simulink model "vip_ut"  (Simulink 8.1)
settings: Solver=FixedStepDiscrete  StartTime=0.0  StopTime=10.0  FixedStep=5E-3  RelTol=1e-3
libraries: siltestlib x17, idiada_lib x7, vip x1
settings Model: Creator=xsellart  LastModifiedBy=AT015555
settings DataIOCC: SignalLoggingSaveFormat=Dataset
settings OptimizationCC: ExpressionDepthLimit=128
settings DebuggingCC: FcnCallInpInsideContextMsg=EnableAllAsError
settings GRTTargetCC: CombineOutputUpdateFcns=on  GRTInterface=off

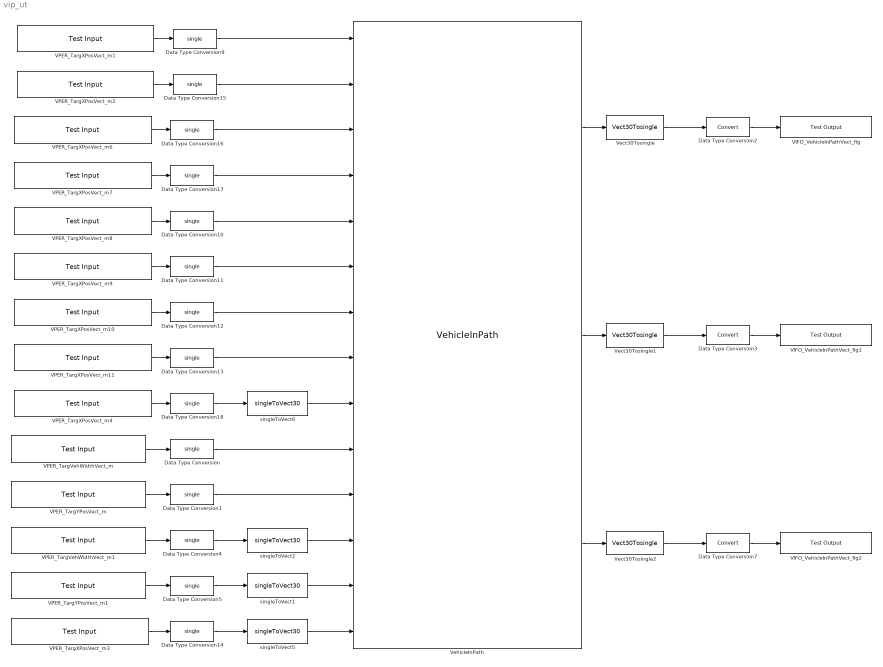
== system vip_ut ==
  Data Type Conversion{,1,4..5,9..18} (14 alike) : DataTypeConversion  OutDataTypeStr=single
  Data Type Conversion2 : DataTypeConversion
  Data Type Conversion3 : DataTypeConversion
  Data Type Conversion7 : DataTypeConversion
  VIFO_VehicleInPathVect_flg : siltestlib/Test Output  varname=VIFO_FCWVehInPathVect30_flg  sampletime=-1
  VIFO_VehicleInPathVect_flg1 : siltestlib/Test Output  varname=VIFO_AEBVehInPathVect30_flg  sampletime=-1
  VIFO_VehicleInPathVect_flg2 : siltestlib/Test Output  varname=VIFO_ACCVehInPathVect30_flg  sampletime=-1
  VPER_TargVehWidthVect_m : siltestlib/Test Input  varname=VDINR_YawRate_degps  sampletime=-1
  VPER_TargVehWidthVect_m1 : siltestlib/Test Input  varname=VPER_TargVehWidthVect30_m  sampletime=-1
  VPER_TargXPosVect_m1 : siltestlib/Test Input  varname=VPER_LaneC0L_m  sampletime=0.005
  VPER_TargXPosVect_m10 : siltestlib/Test Input  varname=VPER_LaneC2R_rat  sampletime=0.005
  VPER_TargXPosVect_m11 : siltestlib/Test Input  varname=VPER_LaneC3R_rat  sampletime=0.005
  VPER_TargXPosVect_m2 : siltestlib/Test Input  varname=VPER_LaneC1L_rad  sampletime=0.005
  VPER_TargXPosVect_m3 : siltestlib/Test Input  varname=VPER_TargYPosVect30_m  sampletime=0.005
  VPER_TargXPosVect_m4 : siltestlib/Test Input  varname=VPER_TargIdVect30_num  sampletime=0.005
  VPER_TargXPosVect_m6 : siltestlib/Test Input  varname=VPER_LaneC2L_rat  sampletime=0.005
  VPER_TargXPosVect_m7 : siltestlib/Test Input  varname=VPER_LaneC3L_rat  sampletime=0.005
  VPER_TargXPosVect_m8 : siltestlib/Test Input  varname=VPER_LaneC0R_m  sampletime=0.005
  VPER_TargXPosVect_m9 : siltestlib/Test Input  varname=VPER_LaneC1R_rad  sampletime=0.005
  VPER_TargYPosVect_m : siltestlib/Test Input  varname=VDINR_SteerAngle_deg  sampletime=-1
  VPER_TargYPosVect_m1 : siltestlib/Test Input  varname=VPER_TargXPosVect30_m  sampletime=-1
  Vect30Tosingle : idiada_lib/Vect30Tosingle
  Vect30Tosingle1 : idiada_lib/Vect30Tosingle
  Vect30Tosingle2 : idiada_lib/Vect30Tosingle
  VehicleInPath : vip/VehicleInPath
  singleToVect{1..2,5..6} (4 alike) : idiada_lib/singleToVect30
  wires:
  VPER_TargVehWidthVect_m/1 -> Data Type Conversion/1
  VPER_TargYPosVect_m/1 -> Data Type Conversion1/1
  Vect30Tosingle/1 -> Data Type Conversion2/1
  Data Type Conversion2/1 -> VIFO_VehicleInPathVect_flg/1
  Vect30Tosingle1/1 -> Data Type Conversion3/1
  Data Type Conversion3/1 -> VIFO_VehicleInPathVect_flg1/1
  VehicleInPath/1 -> Vect30Tosingle/1
  VehicleInPath/2 -> Vect30Tosingle1/1
  VPER_TargVehWidthVect_m1/1 -> Data Type Conversion4/1
  VPER_TargYPosVect_m1/1 -> Data Type Conversion5/1
  Data Type Conversion4/1 -> singleToVect2/1
  Data Type Conversion5/1 -> singleToVect1/1
  Vect30Tosingle2/1 -> Data Type Conversion7/1
  Data Type Conversion7/1 -> VIFO_VehicleInPathVect_flg2/1
  VehicleInPath/3 -> Vect30Tosingle2/1
  VPER_TargXPosVect_m1/1 -> Data Type Conversion9/1
  VPER_TargXPosVect_m2/1 -> Data Type Conversion15/1
  VPER_TargXPosVect_m6/1 -> Data Type Conversion16/1
  VPER_TargXPosVect_m7/1 -> Data Type Conversion17/1
  VPER_TargXPosVect_m8/1 -> Data Type Conversion10/1
  VPER_TargXPosVect_m9/1 -> Data Type Conversion11/1
  VPER_TargXPosVect_m10/1 -> Data Type Conversion12/1
  VPER_TargXPosVect_m11/1 -> Data Type Conversion13/1
  Data Type Conversion15/1 -> VehicleInPath/2
  Data Type Conversion13/1 -> VehicleInPath/8
  Data Type Conversion9/1 -> VehicleInPath/1
  Data Type Conversion17/1 -> VehicleInPath/4
  Data Type Conversion16/1 -> VehicleInPath/3
  Data Type Conversion12/1 -> VehicleInPath/7
  Data Type Conversion11/1 -> VehicleInPath/6
  Data Type Conversion10/1 -> VehicleInPath/5
  VPER_TargXPosVect_m3/1 -> Data Type Conversion14/1
  Data Type Conversion14/1 -> singleToVect5/1
  VPER_TargXPosVect_m4/1 -> Data Type Conversion18/1
  Data Type Conversion18/1 -> singleToVect6/1
  singleToVect6/1 -> VehicleInPath/9
  Data Type Conversion/1 -> VehicleInPath/10
  Data Type Conversion1/1 -> VehicleInPath/11
  singleToVect2/1 -> VehicleInPath/12
  singleToVect1/1 -> VehicleInPath/13
  singleToVect5/1 -> VehicleInPath/14
